simulink model "es2_3_all_directions"  (R2024b)
settings: Solver=VariableStepAuto  StartTime=0.0  StopTime=30  RelTol=1e-3
libraries: sharedutil x1, vrlib x1
settings Model: Creator=danie  LastModifiedBy=danie

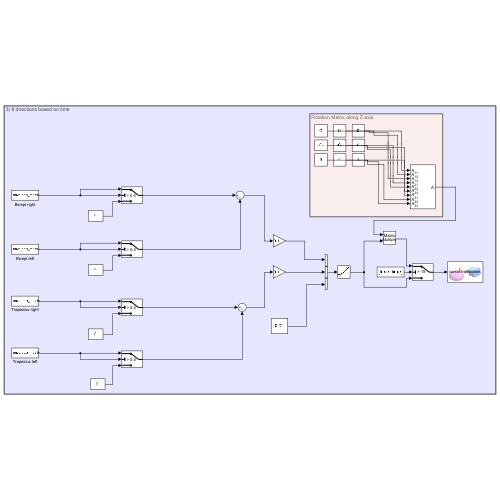
[thumbnail: Simulink's stored preview of the top-level diagram]
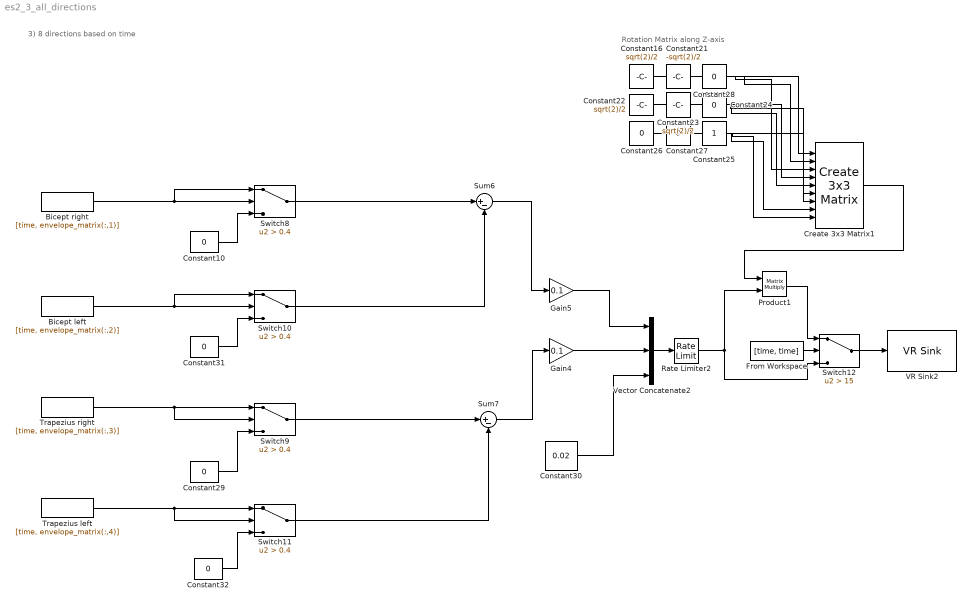
== system es2_3_all_directions ==
  note: 3) 8 directions based on time
  note: Rotation Matrix along Z-axis
  Bicept left : FromWorkspace  VariableName=[time, envelope_matrix(:,2)]
  Bicept right : FromWorkspace  VariableName=[time, envelope_matrix(:,1)]
  Constant{10,24,26..29,31..32} (8 alike) : Constant  Value=0
  Constant16 : Constant  Value=sqrt(2)/2
  Constant21 : Constant  Value=-sqrt(2)/2
  Constant22 : Constant  Value=sqrt(2)/2
  Constant23 : Constant  Value=sqrt(2)/2
  Constant25 : Constant
  Constant30 : Constant  Value=0.02
  Create 3x3 Matrix1 : sharedutil/Create 3x3 Matrix  aMode=aMode
      settings: LibrarySourceBlock=aerolibutil/Create 3x3 Matrix
  From Workspace : FromWorkspace  VariableName=[time, time]
  Gain4 : Gain  Gain=0.1
  Gain5 : Gain  Gain=0.1
  Product1 : Product  Multiplication=Matrix(*)
  Rate Limiter2 : RateLimiter  RisingSlewLimit=0.4  FallingSlewLimit=-0.4  SampleTimeMode=inherited
  Sum6 : Sum  Inputs=|+-
  Sum7 : Sum  Inputs=|+-
  Switch{8..11} (4 alike) : Switch  Criteria=u2 > Threshold  Threshold=0.4  SaturateOnIntegerOverflow=off  InputSameDT=off
  Switch12 : Switch  Criteria=u2 > Threshold  Threshold=15  SaturateOnIntegerOverflow=off  InputSameDT=off
  Trapezius left : FromWorkspace  VariableName=[time, envelope_matrix(:,4)]
  Trapezius right : FromWorkspace  VariableName=[time, envelope_matrix(:,3)]
  VR Sink2 : vrlib/VR Sink  InstantiateOnLoad=on  SampleTime=0.1  ViewEnable=on  RemoteChange=off  RemoteView=off  FieldsWritten=cursor.translation.3.1.1.double  WorldFileName=8_palline_color.wrl  AutoView=off  VideoDimensions=[]  AllowVariableSize=off
  Vector Concatenate2 : Concatenate  NumInputs=3
  wires:
  Constant32/1 -> Switch11/3
  Sum6/1 -> Gain5/1
  Constant23/1 -> Create 3x3 Matrix1/5
  Sum7/1 -> Gain4/1
  Trapezius right/1 -> Switch9/1, Switch9/2
  Switch11/1 -> Sum7/2
  Constant22/1 -> Create 3x3 Matrix1/4
  Bicept right/1 -> Switch8/2, Switch8/1
  From Workspace/1 -> Switch12/2
  Constant25/1 -> Create 3x3 Matrix1/9
  Rate Limiter2/1 -> Switch12/3, Product1/2
  Constant10/1 -> Switch8/3
  Gain4/1 -> Vector Concatenate2/2
  Switch9/1 -> Sum7/1
  Gain5/1 -> Vector Concatenate2/1
  Constant29/1 -> Switch9/3
  Constant31/1 -> Switch10/3
  Switch8/1 -> Sum6/1
  Constant21/1 -> Create 3x3 Matrix1/2
  Constant16/1 -> Create 3x3 Matrix1/1
  Constant27/1 -> Create 3x3 Matrix1/8
  Vector Concatenate2/1 -> Rate Limiter2/1
  Product1/1 -> Switch12/1
  Constant28/1 -> Create 3x3 Matrix1/3
  Switch12/1 -> VR Sink2/1
  Switch10/1 -> Sum6/2
  Trapezius left/1 -> Switch11/1, Switch11/2
  Create 3x3 Matrix1/1 -> Product1/1
  Constant24/1 -> Create 3x3 Matrix1/6
  Constant30/1 -> Vector Concatenate2/3
  Bicept left/1 -> Switch10/1, Switch10/2
  Constant26/1 -> Create 3x3 Matrix1/7
